simulink model "TemplateNoLineal2_2015b"  (R2021a)
settings: Solver=ode4  StartTime=0.0  StopTime=400  FixedStep=0.1  RelTol=1e-3
values from neighbouring files (symbols this model uses):
  u0 = 1    [Problema_3.m]
  x0 = [2, 1, 1]    [Problema_3.m]
  y0 = 1    [Problema_3.m]
libraries: cstblocks x1
settings Model: Creator=aghersin  LastModifiedBy=Santiago
settings SolverCC: AlgebraicLoopSolver=TrustRegion
settings DataIOCC: ReturnWorkspaceOutputs=off
settings OptimizationCC: LifeSpan=inf
settings DebuggingCC: SFExecutionAtInitializationDiag=none  SFMachineParentedDataDiag=warning  ArithmeticOperatorsInVariantConditions=warning
settings SFSimCC: SimUseLocalCustomCode=off  CustomCodeUndefinedFunction=UseInterfaceOnly
settings RTWCC: RTWUseLocalCustomCode=off
settings CodeAppCC: StateflowObjectComments=on

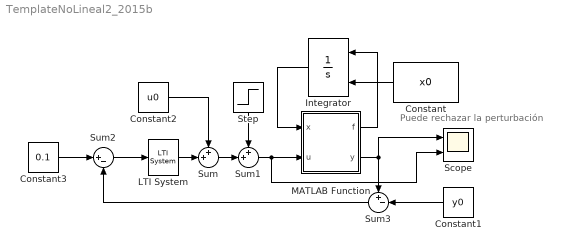
== system TemplateNoLineal2_2015b ==
  note: Puede rechazar la perturbación
  Constant : Constant  Value=x0
  Constant1 : Constant  Value=y0
  Constant2 : Constant  Value=u0
  Constant3 : Constant  Value=0.1
  Integrator : Integrator  InitialConditionSource=external
  LTI System : cstblocks/LTI System  sys=C_dig  IC=[]
  MATLAB Function : MATLAB Function  TreatAsAtomicUnit=on
  Scope : Scope  NumInputPorts=2
  Step : Step  Time=100  After=0.1  SampleTime=0
  Sum : Sum  Inputs=++|
  Sum1 : Sum  Inputs=++|
  Sum2 : Sum  Inputs=|+-
  Sum3 : Sum  Inputs=+-|
  wires:
  Integrator/1 -> MATLAB Function/1(x)
  MATLAB Function/1(f) -> Integrator/1
  Constant/1 -> Integrator/2
  MATLAB Function/2(y) -> Sum3/1, Scope/1
  Constant1/1 -> Sum3/2
  Constant2/1 -> Sum/1
  Sum2/1 -> LTI System/1
  Constant3/1 -> Sum2/1
  Sum3/1 -> Sum2/2
  LTI System/1 -> Sum/2
  Sum/1 -> Sum1/2
  Sum1/1 -> Scope/2, MATLAB Function/2(u)
  Step/1 -> Sum1/1

== matlab function TemplateNoLineal2_2015b/MATLAB Function ==
  data: x input; u input; f output; y output
function [f,y] = fcn(x,u)

p = 0.02;
f1 = (-sqrt(x(1) - x(2)) + x(3) )/x(1)^2;
f2 = (sqrt( x(1) - x(2) ) - sqrt( x(2)) )/x(2)^2;
f3 = -p * x(3) + p * u;
f=[f1; f2; f3];

y=x(2);
